simulink model "gm_untitled1"  (R2024b)
settings: Solver=FixedStepDiscrete  StartTime=0.0  StopTime=10.0  FixedStep=1  RelTol=1e-3
undefined symbols (not defined in the file): jsin
settings Model: Creator=BUVANAPATHI K  LastModifiedBy=yeager
settings OptimizationCC: BlockReduction=off  ConditionallyExecuteInputs=off  DefaultParameterBehavior=Inlined
settings DebuggingCC: AlgebraicLoopMsg=error  InheritedTsInSrcMsg=none
settings HardwareCC: ProdBitPerPointer=32  ProdBitPerSizeT=32  ProdBitPerPtrDiffT=32  ProdLargestAtomicFloat=None  ProdIntDivRoundTo=Undefined  ProdEndianess=Unspecified  ProdWordSize=32  ProdHWDeviceType=ASIC/FPGA->ASIC/FPGA  TargetBitPerLong=64  TargetBitPerPointer=64  TargetBitPerSizeT=64  TargetBitPerPtrDiffT=64  TargetLongLongMode=on  TargetIntDivRoundTo=Zero  TargetEndianess=LittleEndian  TargetWordSize=64  TargetHWDeviceType=Custom Processor->MATLAB Host Computer  ProdEqTarget=off

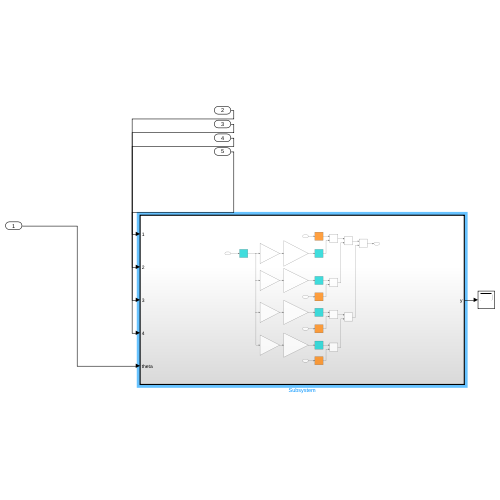
[thumbnail: Simulink's stored preview of the top-level diagram]
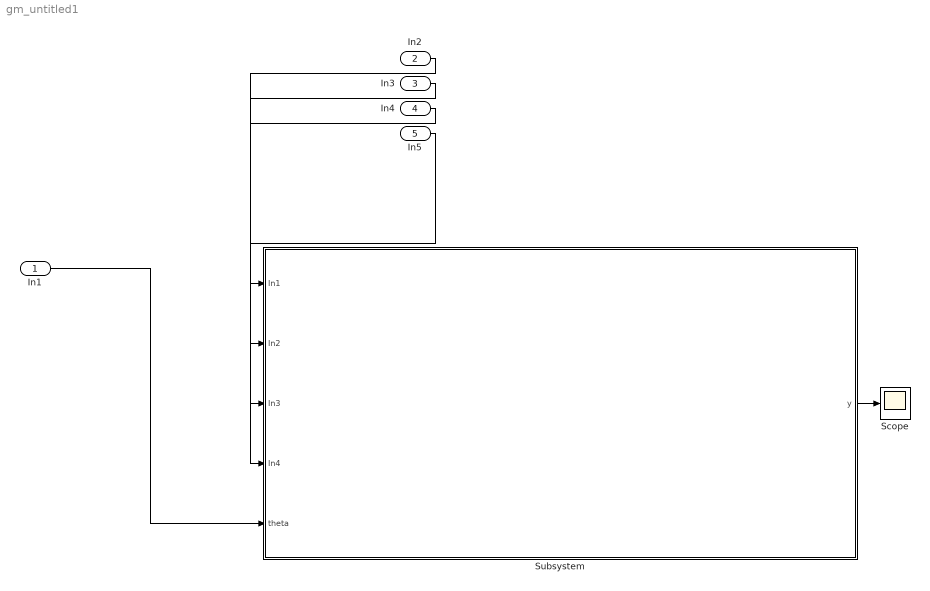
== system gm_untitled1 ==
  In1 : Inport  OutDataTypeStr=fixdt(1,16,12)
  In2 : Inport  Port=2  OutDataTypeStr=fixdt(1,16,12)
  In3 : Inport  Port=3  OutDataTypeStr=fixdt(1,16,12)
  In4 : Inport  Port=4  OutDataTypeStr=fixdt(1,16,12)
  In5 : Inport  Port=5  OutDataTypeStr=fixdt(1,16,12)
  Scope : Scope
  Subsystem : Subsystem  TreatAsAtomicUnit=on
  wires:
  Subsystem/1(y) -> Scope/1
  In1/1 -> Subsystem/5(theta)
  In5/1 -> Subsystem/4(In4)
  In4/1 -> Subsystem/3(In3)
  In3/1 -> Subsystem/2(In2)
  In2/1 -> Subsystem/1(In1)

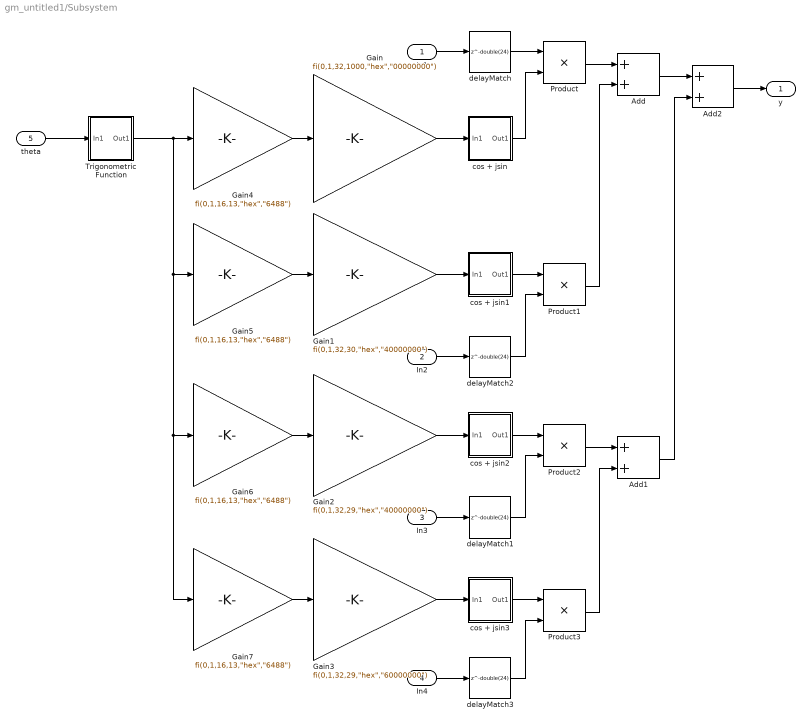
== system gm_untitled1/Subsystem ==
  In1 : Inport  OutDataTypeStr=fixdt(1, 16, 12)  PortDimensions=1  SampleTime=1
      settings: SignalType=complex
  In2 : Inport  Port=2  OutDataTypeStr=fixdt(1, 16, 12)  PortDimensions=1  SampleTime=1
      settings: SignalType=complex
  In3 : Inport  Port=3  OutDataTypeStr=fixdt(1, 16, 12)  PortDimensions=1  SampleTime=1
      settings: SignalType=complex
  In4 : Inport  Port=4  OutDataTypeStr=fixdt(1, 16, 12)  PortDimensions=1  SampleTime=1
      settings: SignalType=complex
  theta : Inport  Port=5  OutDataTypeStr=fixdt(1, 16, 12)  PortDimensions=1  SampleTime=1
  Add : Sum  OutDataTypeStr=fixdt(1, 16, 12)  AccumDataTypeStr=fixdt(1, 16, 12)  SampleTime=1
  Add1 : Sum  OutDataTypeStr=fixdt(1, 16, 12)  AccumDataTypeStr=fixdt(1, 16, 12)  SampleTime=1
  Add2 : Sum  OutDataTypeStr=fixdt(1, 16, 12)  AccumDataTypeStr=fixdt(1, 16, 12)  SampleTime=1
  Gain : Gain  Gain="fi(0,1,32,1000,\"hex\",\"00000000\")"  ParamDataTypeStr=fixdt(1, 32, 1000)  OutDataTypeStr=fixdt(1, 64, 1027)  SampleTime=1
  Gain1 : Gain  Gain="fi(0,1,32,30,\"hex\",\"40000000\")"  ParamDataTypeStr=fixdt(1, 32, 30)  OutDataTypeStr=fixdt(1, 64, 57)  SampleTime=1
  Gain2 : Gain  Gain="fi(0,1,32,29,\"hex\",\"40000000\")"  ParamDataTypeStr=fixdt(1, 32, 29)  OutDataTypeStr=fixdt(1, 64, 56)  SampleTime=1
  Gain3 : Gain  Gain="fi(0,1,32,29,\"hex\",\"60000000\")"  ParamDataTypeStr=fixdt(1, 32, 29)  OutDataTypeStr=fixdt(1, 64, 56)  SampleTime=1
  Gain{4..7} (4 alike) : Gain  Gain="fi(0,1,16,13,\"hex\",\"6488\")"  ParamDataTypeStr=fixdt(1, 16, 13)  OutDataTypeStr=fixdt(1, 32, 27)  SampleTime=1
  Product{,1..3} (4 alike) : Product  Inputs=**  OutDataTypeStr=fixdt(1, 16, 12)  SampleTime=1
  Trigonometric Function : Subsystem
  cos + jsin : Subsystem
  cos + jsin1 : Subsystem
  cos + jsin2 : Subsystem
  cos + jsin3 : Subsystem
  delayMatch{,1..3} (4 alike) : Delay  DelayLength=double(24)  InitialCondition=0  SampleTime=1
  y : Outport  SampleTime=1
  wires:
  Gain7/1 -> Gain3/1
  delayMatch3/1 -> Product3/2
  theta/1 -> Trigonometric Function/1(In1)
  Gain/1 -> cos + jsin/1(In1)
  Trigonometric Function/1(Out1) -> Gain7/1, Gain6/1, Gain5/1, Gain4/1
  Gain6/1 -> Gain2/1
  In1/1 -> delayMatch/1
  Gain4/1 -> Gain/1
  Gain5/1 -> Gain1/1
  Gain1/1 -> cos + jsin1/1(In1)
  delayMatch2/1 -> Product1/2
  In2/1 -> delayMatch2/1
  Gain2/1 -> cos + jsin2/1(In1)
  In3/1 -> delayMatch1/1
  Gain3/1 -> cos + jsin3/1(In1)
  In4/1 -> delayMatch3/1
  delayMatch/1 -> Product/1
  cos + jsin1/1(Out1) -> Product1/1
  cos + jsin/1(Out1) -> Product/2
  cos + jsin3/1(Out1) -> Product3/1
  cos + jsin2/1(Out1) -> Product2/1
  Add/1 -> Add2/1
  Product2/1 -> Add1/1
  delayMatch1/1 -> Product2/2
  Product/1 -> Add/1
  Product1/1 -> Add/2
  Product3/1 -> Add1/2
  Add1/1 -> Add2/2
  Add2/1 -> y/1

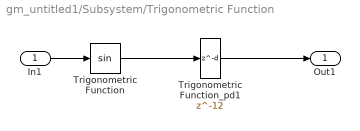
== system gm_untitled1/Subsystem/Trigonometric Function ==
  In1 : Inport
  Trigonometric Function : Trigonometry  ApproximationMethod=CORDIC
  Trigonometric Function_pd1 : Delay  DelayLength=12
  Out1 : Outport
  wires:
  In1/1 -> Trigonometric Function/1
  Trigonometric Function_pd1/1 -> Out1/1
  Trigonometric Function/1 -> Trigonometric Function_pd1/1

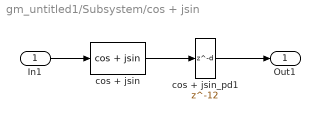
== system gm_untitled1/Subsystem/cos + jsin ==
  In1 : Inport
  cos + jsin : Trigonometry  Operator=cos + jsin  ApproximationMethod=CORDIC
  cos + jsin_pd1 : Delay  DelayLength=12
  Out1 : Outport
  wires:
  In1/1 -> cos + jsin/1
  cos + jsin_pd1/1 -> Out1/1
  cos + jsin/1 -> cos + jsin_pd1/1

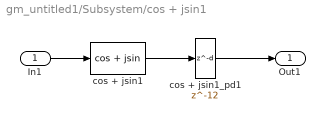
== system gm_untitled1/Subsystem/cos + jsin1 ==
  In1 : Inport
  cos + jsin1 : Trigonometry  Operator=cos + jsin  ApproximationMethod=CORDIC
  cos + jsin1_pd1 : Delay  DelayLength=12
  Out1 : Outport
  wires:
  In1/1 -> cos + jsin1/1
  cos + jsin1_pd1/1 -> Out1/1
  cos + jsin1/1 -> cos + jsin1_pd1/1

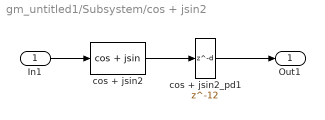
== system gm_untitled1/Subsystem/cos + jsin2 ==
  In1 : Inport
  cos + jsin2 : Trigonometry  Operator=cos + jsin  ApproximationMethod=CORDIC
  cos + jsin2_pd1 : Delay  DelayLength=12
  Out1 : Outport
  wires:
  cos + jsin2_pd1/1 -> Out1/1
  cos + jsin2/1 -> cos + jsin2_pd1/1
  In1/1 -> cos + jsin2/1

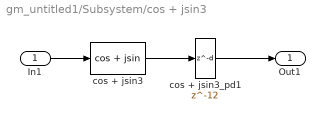
== system gm_untitled1/Subsystem/cos + jsin3 ==
  In1 : Inport
  cos + jsin3 : Trigonometry  Operator=cos + jsin  ApproximationMethod=CORDIC
  cos + jsin3_pd1 : Delay  DelayLength=12
  Out1 : Outport
  wires:
  cos + jsin3_pd1/1 -> Out1/1
  cos + jsin3/1 -> cos + jsin3_pd1/1
  In1/1 -> cos + jsin3/1
